simulink model "PlantaeRealimentacaoPadrao"  (R2019a)
settings: Solver=VariableStepAuto  StartTime=0.0  StopTime=10  RelTol=1e-3
undefined symbols (not defined in the file): A, B, C, K
settings Model: Creator=Cliente  LastModifiedBy=Cliente

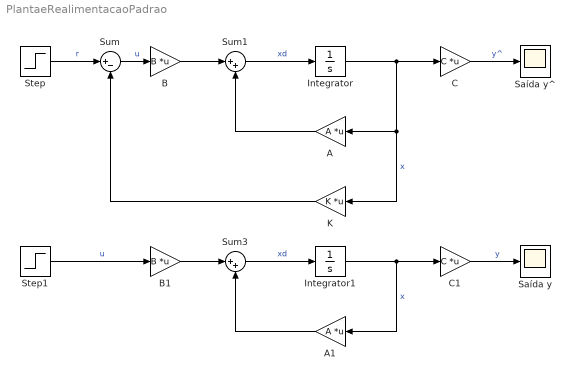
== system PlantaeRealimentacaoPadrao ==
  A : Gain  Gain=A  Multiplication=Matrix(K*u) (u vector)
  A1 : Gain  Gain=A  Multiplication=Matrix(K*u) (u vector)
  B : Gain  Gain=B  Multiplication=Matrix(K*u)
  B1 : Gain  Gain=B  Multiplication=Matrix(K*u)
  C : Gain  Gain=C  Multiplication=Matrix(K*u) (u vector)
  C1 : Gain  Gain=C  Multiplication=Matrix(K*u) (u vector)
  Integrator : Integrator
  Integrator1 : Integrator
  K : Gain  Gain=K  Multiplication=Matrix(K*u) (u vector)
  Saída y : Scope
  Saída y^ : Scope
  Step : Step  Time=0  SampleTime=0
  Step1 : Step  Time=0  SampleTime=0
  Sum : Sum  Inputs=|+-
  Sum1 : Sum  Inputs=|++
  Sum3 : Sum  Inputs=|++
  wires:
  Integrator/1 -> K/1, A/1, C/1  "x"
  Sum1/1 -> Integrator/1  "xd"
  B/1 -> Sum1/1
  Sum/1 -> B/1  "u"
  Step/1 -> Sum/1  "r"
  A/1 -> Sum1/2
  K/1 -> Sum/2
  Integrator1/1 -> A1/1, C1/1  "x"
  Sum3/1 -> Integrator1/1  "xd"
  A1/1 -> Sum3/2
  Step1/1 -> B1/1  "u"
  B1/1 -> Sum3/1
  C/1 -> Saída y^/1  "y^"
  C1/1 -> Saída y/1  "y"
